simulink model "opInvDyn"  (R2021b)
settings: Solver=VariableStepAuto  StartTime=0.0  StopTime=3  RelTol=1e-3
undefined symbols (not defined in the file): Kd, Kp
libraries: robotcorelib x1, simulink x1
settings Model: Creator=fabio  LastModifiedBy=buse

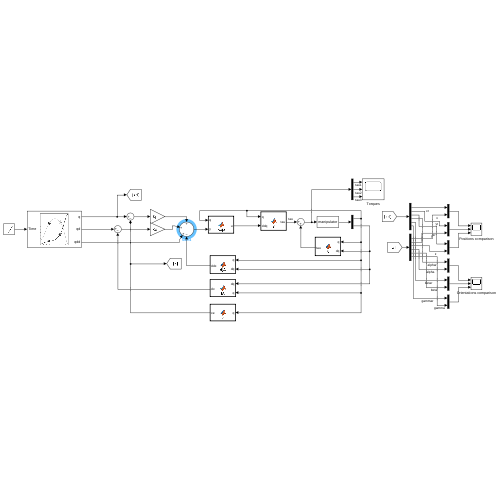
[thumbnail: Simulink's stored preview of the top-level diagram]
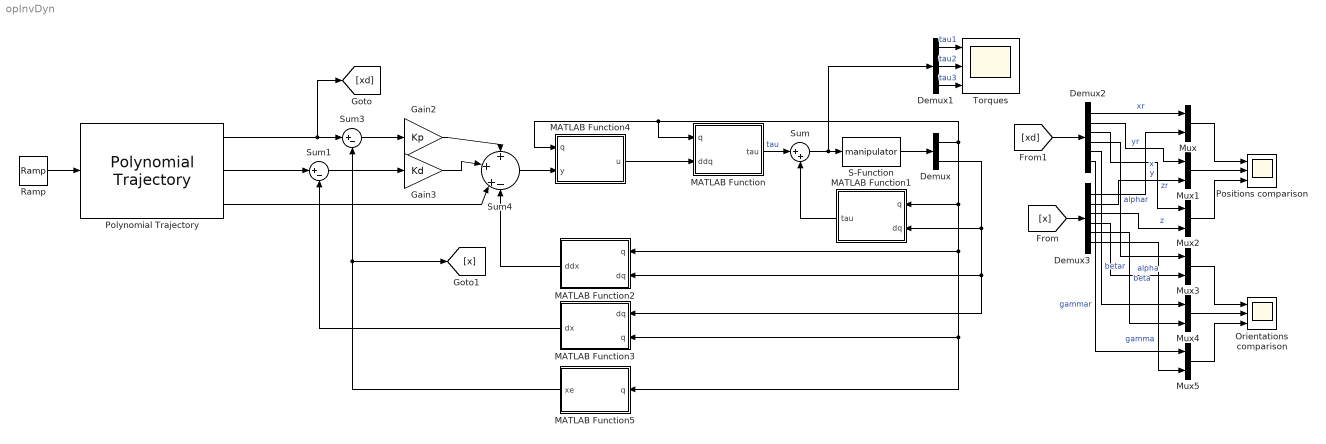
== system opInvDyn ==
  Demux : Demux  Outputs=2
  Demux1 : Demux  Outputs=3
  Demux2 : Demux  Outputs=6
  Demux3 : Demux  Outputs=6
  Gain2 : Gain  Gain=Kp
  Gain3 : Gain  Gain=Kd
  MATLAB Function : MATLAB Function  TreatAsAtomicUnit=on
  MATLAB Function1 : MATLAB Function  TreatAsAtomicUnit=on
  MATLAB Function2 : MATLAB Function  TreatAsAtomicUnit=on
  MATLAB Function3 : MATLAB Function  TreatAsAtomicUnit=on
  MATLAB Function4 : MATLAB Function  TreatAsAtomicUnit=on
  MATLAB Function5 : MATLAB Function  TreatAsAtomicUnit=on
  Mux{,1..5} (6 alike) : Mux  Inputs=2
  Orientations comparison : Scope  NumInputPorts=3
  Polynomial Trajectory : robotcorelib/Polynomial Trajectory  WaypointSource=Internal  Waypoints=op_wpts  TimePoints=time  TimeInterval=[ 1, 4 ]  Method=Quintic Polynomial  ParameterSource=Internal  VelocityBoundaryCondition=velBound  AccelerationBoundaryCondition=accBound  SimulateUsing=Interpreted execution
  Positions comparison : Scope  NumInputPorts=3
  Ramp : simulink/Sources/Ramp  slope=1  start=0  InitialOutput=0
  S-Function : S-Function  FunctionName=manipulator  Parameters=robot  SFunctionDeploymentMode=off  EnableBusSupport=off
  Sum : Sum  Inputs=|++
  Sum1 : Sum  Inputs=|+-
  Sum3 : Sum  Inputs=|+-
  Sum4 : Sum  Inputs=+|+|+-
  Torques : Scope  NumInputPorts=3
  wires:
  Sum3/1 -> Gain2/1
  S-Function/1 -> Demux/1
  Demux/1 -> MATLAB Function3/2(q), MATLAB Function5/1(q), MATLAB Function2/1(q), MATLAB Function1/1(q), MATLAB Function4/1(q), MATLAB Function/1(q)
  Sum1/1 -> Gain3/1
  Demux/2 -> MATLAB Function3/1(dq), MATLAB Function2/2(dq), MATLAB Function1/2(dq)
  Sum/1 -> Demux1/1, S-Function/1
  MATLAB Function/1(tau) -> Sum/1  "tau"
  MATLAB Function1/1(tau) -> Sum/2
  Ramp/1 -> Polynomial Trajectory/1
  Polynomial Trajectory/1 -> [xd], Sum3/1
  Polynomial Trajectory/2 -> Sum1/1
  Demux1/1 -> Torques/1  "tau1"
  Demux1/2 -> Torques/2  "tau2"
  Demux1/3 -> Torques/3  "tau3"
  MATLAB Function5/1(xe) -> [x], Sum3/2
  MATLAB Function3/1(dx) -> Sum1/2
  Sum4/1 -> MATLAB Function4/2(y)
  MATLAB Function4/1(u) -> MATLAB Function/2(ddq)
  Gain2/1 -> Sum4/1
  Gain3/1 -> Sum4/2
  Polynomial Trajectory/3 -> Sum4/3
  MATLAB Function2/1(ddx) -> Sum4/4
  [x] -> Demux3/1
  Mux4/1 -> Orientations comparison/2
  [xd] -> Demux2/1
  Demux2/5 -> Mux4/1  "betar"
  Demux3/6 -> Mux5/2  "gamma"
  Demux3/5 -> Mux4/2  "beta"
  Demux2/2 -> Mux1/1  "yr"
  Mux1/1 -> Positions comparison/2
  Demux2/1 -> Mux/1  "xr"
  Demux2/6 -> Mux5/1  "gammar"
  Demux3/2 -> Mux1/2  "y"
  Mux3/1 -> Orientations comparison/1
  Demux3/4 -> Mux3/2  "alpha"
  Mux5/1 -> Orientations comparison/3
  Demux2/3 -> Mux2/1  "zr"
  Mux2/1 -> Positions comparison/3
  Demux3/1 -> Mux/2  "x"
  Demux2/4 -> Mux3/1  "alphar"
  Mux/1 -> Positions comparison/1
  Demux3/3 -> Mux2/2  "z"

== matlab function opInvDyn/MATLAB Function1 ==
  data: q input size=3; tau output; dq input size=3
function tau = N(q, dq)
    q1 = q(1); q2 = q(2); q3 = q(3);
    dq1 = dq(1); dq2 = dq(2); dq3 = dq(3);
    tau = [dq3*(0.03923*cos(q3)*dq3^2 - 0.5*dq1*(0.0474*sin(2.0*q3) + 0.05885*sin(q3) + 0.1962*q2*sin(q3))*dq3) - 1.0*dq1*(0.5*dq3^2*(0.0474*sin(2.0*q3) + 0.05885*sin(q3) + 0.1962*q2*sin(q3)) - 0.5*dq2^2*(3.098*q2 + 0.1962*cos(q3) + 0.7099)) + 0.5*dq1*dq2^2*(3.098*q2 + 0.1962*cos(q3) + 0.7099);
        0.5*dq1^2*dq2*(3.098*q2 + 0.1962*cos(q3) + 0.7099);
        0.9621*cos(q3) + dq1*(0.03923*cos(q3)*dq3^2 - 0.5*dq1*(0.0474*sin(2.0*q3) + 0.05885*sin(q3) + 0.1962*q2*sin(q3))*dq3)];
end

== matlab function opInvDyn/MATLAB Function ==
  data: q input size=3; tau output; ddq input size=3
function tau = B(q, ddq)
    q1 = q(1); q2 = q(2); q3 = q(3);
        B = [0.7099*q2 + 0.05885*cos(q3) + 0.0474*cos(q3)^2 + 0.1962*q2*cos(q3) + 1.549*q2^2 + 0.496,          -0.6196,  0.03923*sin(q3);
            -0.6196,            1.549, -0.09808*sin(q3);
     0.03923*sin(q3), -0.09808*sin(q3),          0.04757];
    tau = B*ddq;

== matlab function opInvDyn/MATLAB Function2 ==
  data: q input; dq input; ddx output
function ddx = dJA(q,dq)
    q1 = q(1); q2 = q(2); q3 = q(3);
    dq1 = dq(1); dq2 = dq(2); dq3 = dq(3);
    dJA =[dq2*cos(q1) - (2*dq1*cos(q1))/5 - (3*dq1*sin(q1))/10 - dq1*sin(q1)*q2 - (6*dq1*cos(q3)*sin(q1))/25 - (6*dq3*cos(q1)*sin(q3))/25, dq1*cos(q1), - (6*dq1*cos(q1)*sin(q3))/25 - (6*dq3*cos(q3)*sin(q1))/25;
(3*dq1*cos(q1))/10 - (2*dq1*sin(q1))/5 + dq2*sin(q1) + (6*dq1*cos(q1)*cos(q3))/25 - (6*dq3*sin(q1)*sin(q3))/25 + dq1*cos(q1)*q2, dq1*sin(q1),   (6*dq3*cos(q1)*cos(q3))/25 - (6*dq1*sin(q1)*sin(q3))/25;
             0,              0,                                                -(6*dq3*sin(q3))/25;
             0,              0,                                                                     0;
             0,              0,                                                                     0;
             0,              0,                                                                     0];
    ddx = dJA*dq;

== matlab function opInvDyn/MATLAB Function3 ==
  data: dq input; dx output; q input
function dx = JA(dq, q)
    q1 = q(1); q2 = q(2); q3 = q(3);
    JA =[(3*cos(q1))/10 - (2*sin(q1))/5 + (6*cos(q1)*cos(q3))/25 + q2*cos(q1),  sin(q1), -(6*sin(q1)*sin(q3))/25;
        (2*cos(q1))/5 + (3*sin(q1))/10 + (6*cos(q3)*sin(q1))/25 + q2*sin(q1), -cos(q1),  (6*cos(q1)*sin(q3))/25;
        0,        0,          (6*cos(q3))/25;
        1,        0,                       0;
        0,        0,                      -1;
        0,        0,                       0]; 
    dx = JA*dq;

== matlab function opInvDyn/MATLAB Function4 ==
  data: q input; y input; u output
function u = invJA(q,y)
    q1 = q(1); q2 = q(2); q3 = q(3);
    JAinv = [                                                                                                                                            (50*cos(q1)*(50*q2 + 12*cos(q3) + 15))/(1500*q2 + 360*cos(q3) + 144*cos(q3)^2 + 1200*q2*cos(q3) + 2500*q2^2 + 2725),                                                                                                                                              (50*sin(q1)*(50*q2 + 12*cos(q3) + 15))/(1500*q2 + 360*cos(q3) + 144*cos(q3)^2 + 1200*q2*cos(q3) + 2500*q2^2 + 2725),                                   0, 2500/(1500*q2 + 360*cos(q3) + 144*cos(q3)^2 + 1200*q2*cos(q3) + 2500*q2^2 + 2725),                                  0, 0;
(300*cos(q1) + 2725*sin(q1) + 240*cos(q1)*cos(q3) + 2500*q2^2*sin(q1) + 360*cos(q3)*sin(q1) + 144*cos(q3)^2*sin(q1) + 1000*q2*cos(q1) + 1500*q2*sin(q1) + 1200*q2*cos(q3)*sin(q1))/(1500*q2 + 360*cos(q3) + 144*cos(q3)^2 + 1200*q2*cos(q3) + 2500*q2^2 + 2725), -(2725*cos(q1) - 300*sin(q1) + 2500*q2^2*cos(q1) + 360*cos(q1)*cos(q3) - 240*cos(q3)*sin(q1) + 144*cos(q1)*cos(q3)^2 + 1500*q2*cos(q1) - 1000*q2*sin(q1) + 1200*q2*cos(q1)*cos(q3))/(1500*q2 + 360*cos(q3) + 144*cos(q3)^2 + 1200*q2*cos(q3) + 2500*q2^2 + 2725), (18*sin(2*q3))/(18*cos(2*q3) + 643), 1000/(1500*q2 + 360*cos(q3) + 144*cos(q3)^2 + 1200*q2*cos(q3) + 2500*q2^2 + 2725), (150*sin(q3))/(36*sin(q3)^2 - 661), 0;
                                                                                                                                                                                                                                                              0,                                                                                                                                                                                                                                                                0,  (150*cos(q3))/(36*cos(q3)^2 + 625),                                                                                 0,           625/(36*sin(q3)^2 - 661), 0];
 
    u = JAinv*y;

== matlab function opInvDyn/MATLAB Function5 ==
  data: q input size=3; xe output size=6
function xe = k(q)
    q1 = q(1); q2 = q(2); q3 = q(3);
    % Direct kinematics
    xe = [(2*cos(q1))/5 + (3*sin(q1))/10 + (6*cos(q3)*sin(q1))/25 + q2*sin(q1);
         (2*sin(q1))/5 - (3*cos(q1))/10 - (6*cos(q1)*cos(q3))/25 - q2*cos(q1);
         (6*sin(q3))/25 + 3/20;
         q1;
         pi/2 - q3;
         pi/2];
